simulink model "m20222023"  (R2016a)
settings: Solver=VariableStepAuto  StartTime=0.0  StopTime=5  RelTol=1e-3
settings Model: Creator=witkey721  LastModifiedBy=witkey721

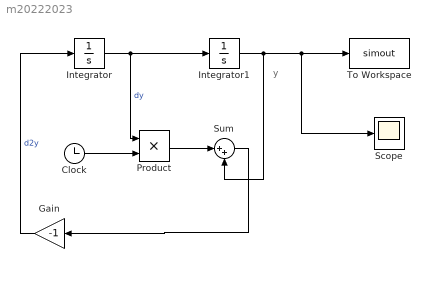
== system m20222023 ==
  note: y
  Clock : Clock
  Gain : Gain  Gain=-1
  Integrator : Integrator  InitialCondition=1
  Integrator1 : Integrator
  Product : Product
  Scope : Scope
  Sum : Sum  Inputs=|++
  To Workspace : ToWorkspace  VariableName=simout  SaveFormat=Timeseries  SampleTime=-1
  wires:
  Integrator/1 -> Product/1, Integrator1/1  "dy"
  Gain/1 -> Integrator/1  "d2y"
  Clock/1 -> Product/2
  Product/1 -> Sum/1
  Integrator1/1 -> Scope/1, To Workspace/1, Sum/2
  Sum/1 -> Gain/1
